simulink model "Grav_VarConst"  (R2016b)
settings: Solver=VariableStepAuto  StartTime=0.0  StopTime=10.0  RelTol=1e-3
undefined symbols (not defined in the file or in its folder): Env
settings Model: Creator=rega0051  LastModifiedBy=rega0051
settings DataIOCC: SaveOutput=off  SignalLogging=off  DSMLogging=off  SaveTime=off

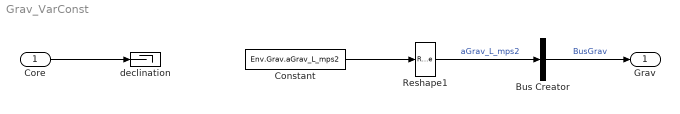
== system Grav_VarConst ==
  Core : Inport  OutDataTypeStr=Bus: BusCore
      settings: AttributesFormatString=%<OutDataTypeStr>
  Bus Creator : BusCreator  Inputs=1  OutDataTypeStr=Bus: BusGrav
      settings: AttributesFormatString=%<OutDataTypeStr>
  Constant : Constant  Value=Env.Grav.aGrav_L_mps2  SampleTime=-1
      settings: AttributesFormatString=%<Value>
  Reshape1 : Reshape  OutputDimensionality=Column vector (2-D)  OutputDimensions=[3,1]
  declination : Terminator
  Grav : Outport  OutDataTypeStr=Bus: BusGrav
      settings: AttributesFormatString=%<OutDataTypeStr>
  wires:
  Constant/1 -> Reshape1/1
  Bus Creator/1 -> Grav/1  "BusGrav"
  Core/1 -> declination/1
  Reshape1/1 -> Bus Creator/1  "aGrav_L_mps2"
